simulink model "test_model"  (R2021a)
settings: Solver=FixedStepAuto  StartTime=0.0  StopTime=[18;]  FixedStep=[0.01;]  RelTol=1e-3
settings Model: Creator=beave  LastModifiedBy=thana
settings SolverCC: AlgebraicLoopSolver=TrustRegion
settings DebuggingCC: SFMachineParentedDataDiag=warning

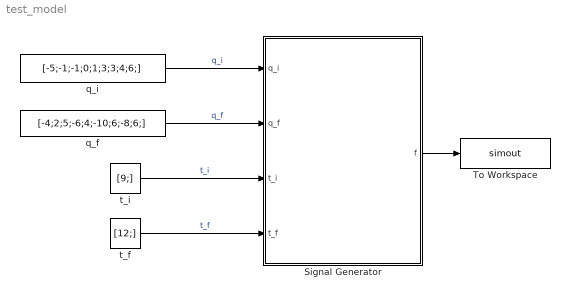
== system test_model ==
  Signal Generator : Subsystem
  To Workspace : ToWorkspace  VariableName=simout  SaveFormat=Timeseries  SampleTime=-1
  q_f : Constant  Value=[-4;2;5;-6;4;-10;6;-8;6;]
  q_i : Constant  Value=[-5;-1;-1;0;1;3;3;4;6;]
  t_f : Constant  Value=[12;]
  t_i : Constant  Value=[9;]
  wires:
  q_i/1 -> Signal Generator/1(q_i)  "q_i"
  q_f/1 -> Signal Generator/2(q_f)  "q_f"
  t_i/1 -> Signal Generator/3(t_i)  "t_i"
  t_f/1 -> Signal Generator/4(t_f)  "t_f"
  Signal Generator/1(f) -> To Workspace/1

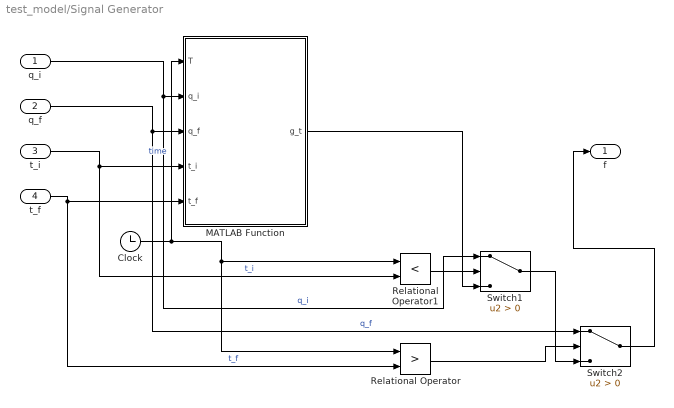
== system test_model/Signal Generator ==
  q_i : Inport
  q_f : Inport  Port=2
  t_i : Inport  Port=3
  t_f : Inport  Port=4
  Clock : Clock
  MATLAB Function : MATLAB Function  TreatAsAtomicUnit=on
  Relational Operator : RelationalOperator  Operator=>  OutDataTypeStr=boolean  RndMeth=Simplest
  Relational Operator1 : RelationalOperator  Operator=<  OutDataTypeStr=boolean  RndMeth=Simplest
  Switch1 : Switch  Criteria=u2 > Threshold
  Switch2 : Switch  Criteria=u2 > Threshold
  f : Outport
  wires:
  Switch2/1 -> f/1
  Switch1/1 -> Switch2/3
  Relational Operator1/1 -> Switch1/2
  t_i/1 -> MATLAB Function/4(t_i), Relational Operator1/2  "t_i"
  q_i/1 -> Switch1/1, MATLAB Function/2(q_i)  "q_i"
  Relational Operator/1 -> Switch2/2
  q_f/1 -> Switch2/1, MATLAB Function/3(q_f)  "q_f"
  Clock/1 -> MATLAB Function/1(T), Relational Operator/1, Relational Operator1/1  "time"
  t_f/1 -> MATLAB Function/5(t_f), Relational Operator/2  "t_f"
  MATLAB Function/1(g_t) -> Switch1/3

== matlab function test_model/Signal Generator/MATLAB Function ==
  data: T input; q_i input; q_f input; t_i input; g_t output; t_f input
function g_t = fcn(T,q_i,q_f,t_i,t_f)
%สร้างตัวแปร C ที่มีขนาดเท่ากับเมทริกซ์ [จำนนวนVectorที่รับเข้ามา x สัมประสิทธิ์]
c = zeros(numel(q_i),4);
%{
สร้างลูปจำนวน numel(q_i) ครั้งเพื่อรันเว็กเตอร์ทุกตัวที่รับค่าเข้ามา
สร้าง RHS ที่เป็นเมทริกซ์ทางด้านขวามือของสมการ
และสร้าง A เป็นเมทริกซ์ทางด้านซ้ายของสมการเพื่อใช้ในการแก้สมการ
ตั้งให้ ac0,ac1,ac2,ac3 มีค่าเท่ากับ A ที่แทนค่าColumnที่ 1,2,3,4
ตามลำดับเพื่อนำไปใช้แก้สมการหาสัมประสิทธิ์โดยสมการ c_x = det(acx) / det(A)
โดยที่ x = {0,1,2,3} เมื่อได้ c แล้ว
เก็บ c ในรูปแบบของ array ด้วย c(i,:) = [c_3 c_2 c_1 c_0];
ในแต่ละลูป และนำ c ไปใช้ในการสร้างสัญญาณที่มี input มากจาก Clock ใน
simulink โดยให้ output เป็น g_t = c(:,4) + c(:,3)*T + c(:,2)*(T.^2) + c(:,1)*(T.^3) ;
เพื่อให้ g_t พลอตค่าออกมาในทุกๆ ROW ในฟังก์ชั่น c
%}
for i = 1:numel(q_i)
    RHS = [q_i(i) ; q_f(i) ; 0 ; 0 ];
    A = [1 t_i (t_i^2) (t_i^3) ; 1 t_f (t_f^2) (t_f^3) ; 0 1 (2*t_i) (3*(t_i^2)) ;  0 1 (2*t_f) (3*(t_f^2))] ;
    ac0 = A ;
    ac0(:,1) = RHS';
    c_0 = det(ac0)/ det(A) ;
    ac1 = A ;
    ac1(:,2) = RHS';
    c_1 = det(ac1)/ det(A) ;
    ac2 = A ;
    ac2(:,3) = RHS';
    c_2 = det(ac2)/ det(A) ;
    ac3 = A ;
    ac3(:,4) = RHS';
    c_3 = det(ac3)/ det(A) ;
    c(i,:) = [c_3 c_2 c_1 c_0];
    g_t = c(:,4) + c(:,3)*T + c(:,2)*(T.^2) + c(:,1)*(T.^3) ;
end
